simulink model "SimulinkHvac_2018a_pso"  (R2021b)
settings: Solver=ode4  StartTime=0.0  StopTime=600  FixedStep=600  RelTol=1e-3
values from neighbouring files (symbols this model uses):
  T_1_0 = T_1    [main_p2.m]
  T_2_0 = T_2    [main_p2.m]
settings Model: SimulationMode=accelerator  Creator=rober  LastModifiedBy=Bruno
settings SolverCC: AlgebraicLoopSolver=TrustRegion
settings DataIOCC: ReturnWorkspaceOutputs=off
settings OptimizationCC: LifeSpan=inf
settings DebuggingCC: SFMachineParentedDataDiag=warning  ArithmeticOperatorsInVariantConditions=warning
settings SFSimCC: CustomCodeUndefinedFunction=UseInterfaceOnly
settings CodeAppCC: StateflowObjectComments=on

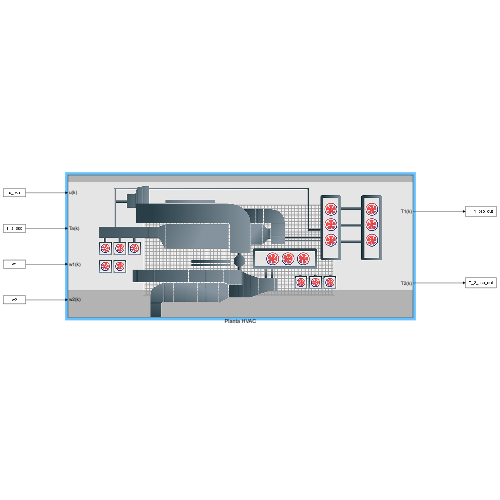
[thumbnail: Simulink's stored preview of the top-level diagram]
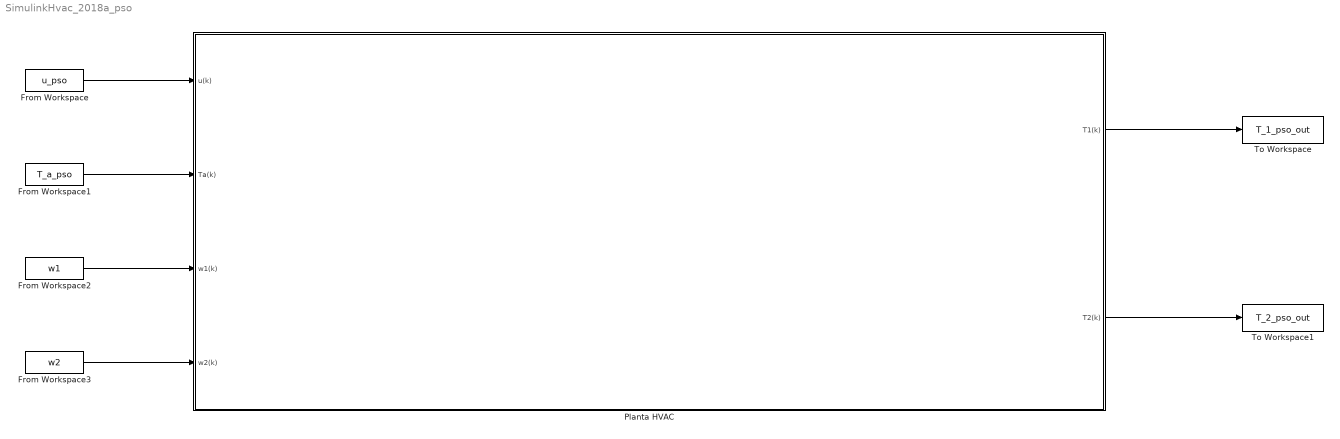
== system SimulinkHvac_2018a_pso ==
  From Workspace : FromWorkspace  VariableName=u_pso  SampleTime=-1
  From Workspace1 : FromWorkspace  VariableName=T_a_pso  SampleTime=-1
  From Workspace2 : FromWorkspace  VariableName=w1  SampleTime=-1
  From Workspace3 : FromWorkspace  VariableName=w2  SampleTime=-1
  Planta HVAC : Subsystem
      mask Display: image('Planta_HVAC.jpg')
  To Workspace : ToWorkspace  VariableName=T_1_pso_out  SampleTime=-1
  To Workspace1 : ToWorkspace  VariableName=T_2_pso_out  SampleTime=-1
  wires:
  From Workspace/1 -> Planta HVAC/1(u(k))
  From Workspace1/1 -> Planta HVAC/2(Ta(k))
  From Workspace2/1 -> Planta HVAC/3(w1(k))
  From Workspace3/1 -> Planta HVAC/4(w2(k))
  Planta HVAC/1(T1(k)) -> To Workspace/1
  Planta HVAC/2(T2(k)) -> To Workspace1/1

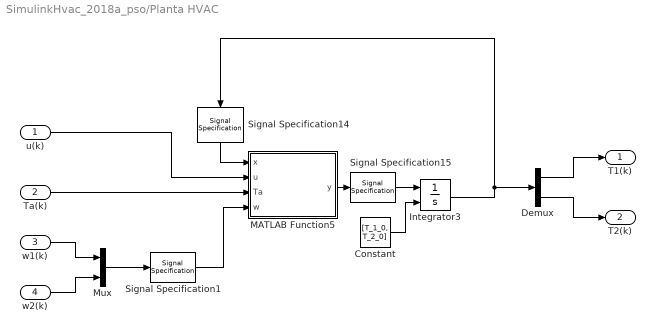
== system SimulinkHvac_2018a_pso/Planta HVAC ==
  u(k) : Inport
  Ta(k) : Inport  Port=2
  w1(k) : Inport  Port=3
  w2(k) : Inport  Port=4
  Constant : Constant  Value=[T_1_0, T_2_0]
  Demux : Demux  Outputs=2
  Integrator3 : Integrator  InitialConditionSource=external  InitialCondition=[10.12;10.12]
  MATLAB Function5 : MATLAB Function  TreatAsAtomicUnit=on
  Mux : Mux  Inputs=2
  Signal Specification1 : SignalSpecification  Dimensions=[2,1]
  Signal Specification14 : SignalSpecification  Dimensions=[2,1]
  Signal Specification15 : SignalSpecification  Dimensions=[2,1]
  T1(k) : Outport
  T2(k) : Outport  Port=2
  wires:
  MATLAB Function5/1(y) -> Signal Specification15/1
  Demux/1 -> T1(k)/1
  u(k)/1 -> MATLAB Function5/2(u)
  Ta(k)/1 -> MATLAB Function5/3(Ta)
  Integrator3/1 -> Demux/1, Signal Specification14/1
  Signal Specification14/1 -> MATLAB Function5/1(x)
  Signal Specification15/1 -> Integrator3/1
  Demux/2 -> T2(k)/1
  Mux/1 -> Signal Specification1/1
  w1(k)/1 -> Mux/1
  w2(k)/1 -> Mux/2
  Signal Specification1/1 -> MATLAB Function5/4(w)
  Constant/1 -> Integrator3/2

== matlab function SimulinkHvac_2018a_pso/Planta HVAC/MATLAB Function5 ==
  data: x input; u input; y output; Ta input; w input
function y = fcn(x,u,Ta,w)
%% Parametros
c1=2.508*10^6;
c2=4.636*10^7;
cp=1012;
R=1.7*10^(-3);
Ra=1.3*10^(-3);
delta=0.7;
DeltaT=13;
%% Constantes
a1=(cp*(1-delta))/c1;
a2=1/(R*c1);
a3=1/(Ra*c1);
a4=(DeltaT*cp)/c1;
a5=1/c1;
a6=1/(R*c2);
a7=1/c2;
%% Calculo del sistema
xdot=zeros(2,1);
xdot(1)=a1*(Ta-x(1))*u+a2*(x(2)-x(1))+a3*(Ta-x(1))+a4*u+a5*w(1);
xdot(2)=a6*(x(1)-x(2))+a7*w(2);
y = xdot;
